simulink model "IEEE_39_bus_steady_state"  (R2021b)
settings: Solver=ode3  StartTime=0.0  StopTime=10  FixedStep=Ts  MaxStep=1/60  RelTol=1e-2  AbsTol=1e-1
PreLoadFcn:
  | Ts=50e-6; ssn_ieee39_params; dec=20;
InitFcn:
  | Ts=50e-6; ssn_ieee39_params; dec=20;
values from neighbouring files (symbols this model uses):
  f = 50    [ssn_ieee39_params_ctrl.m]
  fNom = f    (= 60)    [ssn_ieee39_params_ctrl.m]
  ILR = 5.02    [ssn_ieee39_params_ctrl.m]
  IQMIN = 0.1    [ssn_ieee39_params_ctrl.m]
  ISCLIM = 1    [ssn_ieee39_params_ctrl.m]
  ITFpu = 1.10    (= 1.1)    [ssn_ieee39_params_ctrl.m]
  K = 1    [ssn_ieee39_params_ctrl.m]
  K1 = 1    [ssn_ieee39_params_ctrl.m]
  K2 = 2    [ssn_ieee39_params_ctrl.m]
  KCL = 1.04    [ssn_ieee39_params_ctrl.m]
  KFB = 0    [ssn_ieee39_params_ctrl.m]
  KFF = 1    [ssn_ieee39_params_ctrl.m]
  KFIX = 1    [ssn_ieee39_params_ctrl.m]
  KG = 1    [ssn_ieee39_params_ctrl.m]
  KIA = 59.91    [ssn_ieee39_params_ctrl.m]
  KIOEX = 0.0303    [ssn_ieee39_params_ctrl.m]
  KIUEX = 0.0303    [ssn_ieee39_params_ctrl.m]
  KIUOEX = 1    [ssn_ieee39_params_ctrl.m]
  KIUUEX = 1    [ssn_ieee39_params_ctrl.m]
  KLR = 22.47    [ssn_ieee39_params_ctrl.m]
  KM = 1    [ssn_ieee39_params_ctrl.m]
  KOEL = 0.24    [ssn_ieee39_params_ctrl.m]
  Kp = 1    [ssn_ieee39_params_ctrl.m]
  KPA = 30    [ssn_ieee39_params_ctrl.m]
  KPOEL = 1    [ssn_ieee39_params_ctrl.m]
  KPOEX = 0    [ssn_ieee39_params_ctrl.m]
  KPUEX = 0    [ssn_ieee39_params_ctrl.m]
  KSCALE = 0.319    [ssn_ieee39_params_ctrl.m]
  KUF = 0    [ssn_ieee39_params_ctrl.m]
  KUI = 0.001    [ssn_ieee39_params_ctrl.m]
  KUL = 0.24    [ssn_ieee39_params_ctrl.m]
  s = 10    [ssn_ieee39_params_ctrl.m]
  TA = 0.01    [ssn_ieee39_params_ctrl.m]
  Tadj = 0    [ssn_ieee39_params_ctrl.m]
  taps = [1 1 1.07 1.07 1.009 1.025 1 1.025 1.025 1.025]*1    [ssn_ieee39_params_ctrl.m]
  TF = 0.02    [ssn_ieee39_params_ctrl.m]
  TG = 0.024    [ssn_ieee39_params_ctrl.m]
  TINV = 0    [ssn_ieee39_params_ctrl.m]
  TIT = 0.1    [ssn_ieee39_params_ctrl.m]
  TL_10_11_len = 14    [ssn_ieee39_params_ctrl.m]
  TL_10_13_len = 14    [ssn_ieee39_params_ctrl.m]
  TL_13_14_len = 32    [ssn_ieee39_params_ctrl.m]
  TL_14_15_len = 70    [ssn_ieee39_params_ctrl.m]
  TL_15_16_len = 31.5    [ssn_ieee39_params_ctrl.m]
  TL_16_17_len = 26    [ssn_ieee39_params_ctrl.m]
  TL_16_19_len = 61    [ssn_ieee39_params_ctrl.m]
  TL_16_21_len = 46    [ssn_ieee39_params_ctrl.m]
  TL_16_24_len = 15    [ssn_ieee39_params_ctrl.m]
  TL_17_18_len = 26    [ssn_ieee39_params_ctrl.m]
  TL_17_27_len = 59    [ssn_ieee39_params_ctrl.m]
  TL_1_2_len = 134    [ssn_ieee39_params_ctrl.m]
  TL_1_39_len = 105    [ssn_ieee39_params_ctrl.m]
  TL_21_22_len = 47    [ssn_ieee39_params_ctrl.m]
  TL_22_23_len = 33    [ssn_ieee39_params_ctrl.m]
  TL_24_23_len = 88    [ssn_ieee39_params_ctrl.m]
  TL_25_26_len = 101    [ssn_ieee39_params_ctrl.m]
  TL_26_27_len = 46.5    [ssn_ieee39_params_ctrl.m]
  TL_26_28_len = 151    [ssn_ieee39_params_ctrl.m]
  TL_26_29_len = 200    [ssn_ieee39_params_ctrl.m]
  TL_28_29_len = 48    [ssn_ieee39_params_ctrl.m]
  TL_2_25_len = 28    [ssn_ieee39_params_ctrl.m]
  TL_2_2_len = 49    [ssn_ieee39_params_ctrl.m]
  TL_3_18_len = 42    [ssn_ieee39_params_ctrl.m]
  TL_3_4_len = 53    [ssn_ieee39_params_ctrl.m]
  TL_4_14_len = 33    [ssn_ieee39_params_ctrl.m]
  TL_4_5_len = 32.5    [ssn_ieee39_params_ctrl.m]
  TL_5_6_len = 14    [ssn_ieee39_params_ctrl.m]
  TL_5_8_len = 32    [ssn_ieee39_params_ctrl.m]
  TL_6_11_len = 26.5    [ssn_ieee39_params_ctrl.m]
  TL_6_7_len = 25.5    [ssn_ieee39_params_ctrl.m]
  TL_7_8_len = 15    [ssn_ieee39_params_ctrl.m]
  TL_8_9_len = 93    [ssn_ieee39_params_ctrl.m]
  TL_9_39_len = 136    [ssn_ieee39_params_ctrl.m]
  TOEL = 5.00    (= 5)    [ssn_ieee39_params_ctrl.m]
  TQREF = 0    [ssn_ieee39_params_ctrl.m]
  TQSCL = 0.012    [ssn_ieee39_params_ctrl.m]
  Ts_PMU = 1/1000    (= 0.001)    [ssn_ieee39_params_ctrl.m]
  TU1 = 0    [ssn_ieee39_params_ctrl.m]
  TU2 = 0    [ssn_ieee39_params_ctrl.m]
  TU3 = 0    [ssn_ieee39_params_ctrl.m]
  TU4 = 0    [ssn_ieee39_params_ctrl.m]
  TUL = 0    [ssn_ieee39_params_ctrl.m]
  TUP = 0.050    (= 0.05)    [ssn_ieee39_params_ctrl.m]
  TUQ = .005    (= 0.005)    [ssn_ieee39_params_ctrl.m]
  TUV = 0.2    [ssn_ieee39_params_ctrl.m]
  VAAMAX = VAMAX    (= 7.05)    [ssn_ieee39_params_ctrl.m]
  VAMAX = 7.05    [ssn_ieee39_params_ctrl.m]
  VAMIN = -6.11    [ssn_ieee39_params_ctrl.m]
  VBMAX = 999    [ssn_ieee39_params_ctrl.m]
  VF = 0    [ssn_ieee39_params_ctrl.m]
  VFB = 0    [ssn_ieee39_params_ctrl.m]
  VMMAX = 7.05    [ssn_ieee39_params_ctrl.m]
  VMMIN = -6.11    [ssn_ieee39_params_ctrl.m]
  VOELmax1 = 0.2353    [ssn_ieee39_params_ctrl.m]
  VOELmax2 = 0.0    (= 0)    [ssn_ieee39_params_ctrl.m]
  VOELmin1 = -0.24    [ssn_ieee39_params_ctrl.m]
  VOELmin2 = -1.0    (= -1)    [ssn_ieee39_params_ctrl.m]
  VRMAX = 7.05    [ssn_ieee39_params_ctrl.m]
  VRMIN = -6.11    [ssn_ieee39_params_ctrl.m]
  VSCLmax = 0.20    (= 0.2)    [ssn_ieee39_params_ctrl.m]
  VSCLmin = -0.10    (= -0.1)    [ssn_ieee39_params_ctrl.m]
  VUELmax1 = 1    [ssn_ieee39_params_ctrl.m]
  VUELmax2 = 1    [ssn_ieee39_params_ctrl.m]
  VUELmin1 = -1    [ssn_ieee39_params_ctrl.m]
  VUELmin2 = -1    [ssn_ieee39_params_ctrl.m]
  VUImax = 1    [ssn_ieee39_params_ctrl.m]
  VUImin = -1    [ssn_ieee39_params_ctrl.m]
undefined symbols (not defined in the file or in its folder): D1, Delta, MOV_segment9, powergui
libraries: spsThreePhaseVIMeasurementLib x43, slpidlib x40, op_dpl_lib x32, powerlib_extras x30, simulink_extras x20, spsST2AModel x20, spsThreePhaseParallelRLCLoadLib x20, spsThreePhaseTransformerTwoWindingsLib x13, spsSynchronousMachinepuStandardLib x10, simulink x10, spsPower3phInstantaneousLib x10, spsThreePhasePISectionLineLib x4
(part 15 of 15)

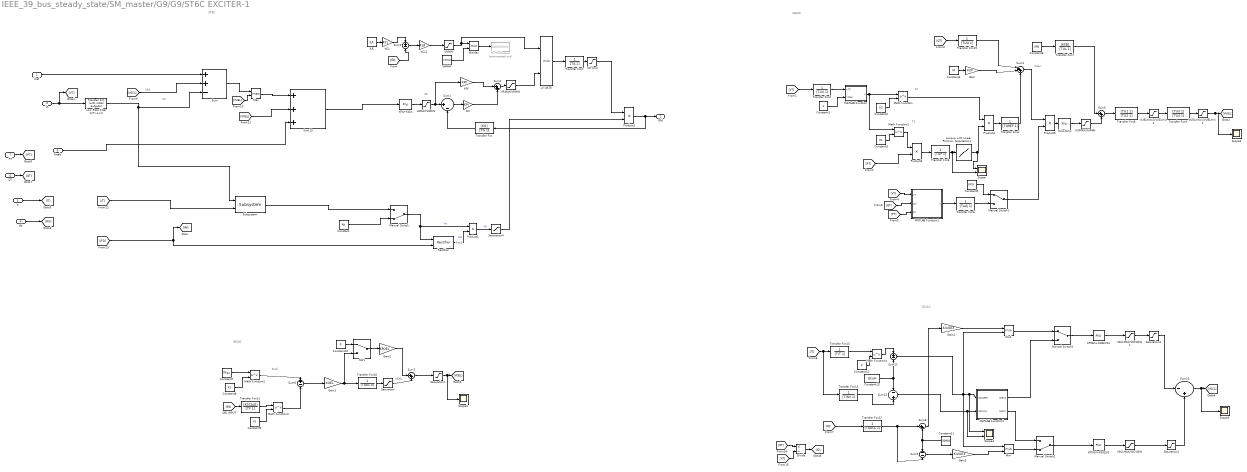
== system IEEE_39_bus_steady_state/SM_master/G9/G9/ST6C EXCITER-1 ==
  note: SCL1C
  note: OEL3C
  note: UEL2C
  note: VR0
  note: Fex0
  note: VA
  note: F2
  note: F1
  note: VUerr
  note: ST6C
  note: IFref
  note: VIOEL
  note: VC
  Vref : Inport
  Vt : Inport  Port=2
  It : Inport  Port=3
  Ifd : Inport  Port=4
  Vstab : Inport  Port=5
  QT : Inport  Port=6
  PT : Inport  Port=7
  Constant : Constant  Value=Kp
  Constant1 : Constant
  Constant10 : Constant  Value=0
  Constant11 : Constant  Value=IQMIN
  Constant12 : Constant  Value=K
  Constant13 : Constant  Value=ISCLIM
  Constant2 : Constant  Value=K2
  Constant3 : Constant  Value=K1
  Constant4 : Constant  Value=VF
  Constant5 : Constant  Value=KFIX
  Constant6 : Constant  Value=VFB
  Constant7 : Constant  Value=ITFpu
  Constant8 : Constant  Value=K1
  Constant9 : Constant  Value=K1
  Divide : Product  Inputs=*/
  Gain : Gain  Gain=KUF
  Gain1 : Gain  Gain=KOEL
  Gain2 : Gain  Gain=KPOEL
  Gain3 : Gain  Gain=KIUUEX
  Gain4 : Gain  Gain=KIUOEX
  ILR : Constant  Value=ILR
  KCL : Gain  Gain=KCL
  KCL1 : Gain  Gain=KLR
  KFF : Gain  Gain=KFF
  KM : Gain  Gain=KM
  KPA+KIA/s : slpidlib/PID Controller  Controller=PI  Form=Parallel  TimeDomain=Continuous-time  UseExternalTs=off  SampleTime=-1  IntegratorMethod=Forward Euler  FilterMethod=Forward Euler  ControllerParametersSource=internal  P=KPA  I=KIA  D=0  UseFilter=on  N=100  TunerSelectOption=Transfer Function Based (PID Tuner App)  InitialConditionSource=internal  InitialConditionForIntegrator=0  InitialConditionForFilter=0  DifferentiatorICPrevScaledInput=0  ExternalReset=none  TrackingMode=off  Kt=1  LimitOutput=off  SatLimitsSource=internal  UpperSaturationLimit=inf  LowerSaturationLimit=-inf  LinearizeAsGain=on  AntiWindupMode=none  Kb=1  POutMin=[]  POutMax=[]  IOutMin=[]  IOutMax=[]  DOutMin=[]  DOutMax=[]  NOutMin=[]  NOutMax=[]  SumOutMin=[]  SumOutMax=[]  SaturationOutMin=[]  SaturationOutMax=[]  PParamMin=[]  PParamMax=[]  IParamMin=[]  IParamMax=[]  DParamMin=[]  DParamMax=[]  NParamMin=[]  NParamMax=[]  KbParamMin=[]  KbParamMax=[]  KtParamMin=[]  KtParamMax=[]  KbOutMin=[]  KbOutMax=[]  KtOutMin=[]  KtOutMax=[]  IntegratorOutMin=[]  IntegratorOutMax=[]  FilterOutMin=[]  FilterOutMax=[]  SumI1OutMin=[]  SumI1OutMax=[]  SumI2OutMin=[]  SumI2OutMax=[]  SumI3OutMin=[]  SumI3OutMax=[]  SumI4OutMin=[]  SumI4OutMax=[]  SumDOutMin=[]  SumDOutMax=[]  DifferentiatorOutMin=[]  DifferentiatorOutMax=[]  FilterDiffOutCoefMin=[]  FilterDiffOutCoefMax=[]  ReciprocalOutMin=[]  ReciprocalOutMax=[]  SumDenOutMin=[]  SumDenOutMax=[]  SumNumOutMin=[]  SumNumOutMax=[]  DivideOutMin=[]  DivideOutMax=[]  UdiffTsProdOutMin=[]  UdiffTsProdOutMax=[]  NTsProdOutMin=[]  NTsProdOutMax=[]  UintegralTsProdOutMin=[]  UintegralTsProdOutMax=[]  UngainTsProdOutMin=[]  UngainTsProdOutMax=[]  FilterDenConstantOutDataTypeStr=Inherit: Inherit via back propagation  FilterDenConstantOutMin=[]  FilterDenConstantOutMax=[]  PCopyOutDataTypeStr=Inherit: Inherit via back propagation  PCopyOutMin=[]  PCopyOutMax=[]  NCopyOutDataTypeStr=Inherit: Inherit via back propagation  NCopyOutMin=[]  NCopyOutMax=[]  IntegratorContinuousStateAttributes=''  IntegratorStateMustResolveToSignalObject=off  IntegratorRTWStateStorageClass=Auto  FilterContinuousStateAttributes=''  FilterStateMustResolveToSignalObject=off  FilterRTWStateStorageClass=Auto  ParallelPVariant=InternalParameters  IdealPVariant=Disabled  IVariant=InternalParameters  DVariant=Disabled  IntegratorVariant=Continuous  SatVariant=Disabled  AWVariant=Passthrough  PCopyVariant=Disabled  TRVariant=Disabled  FdbkBlocksVariant=Forward  IdealPFdbkVariant=Disabled  SatFdbkVariant=Disabled  DerivativeFilterVariant=Disabled  NVariant=Disabled  NCopyVariant=Disabled_SignalSpec  FilterICVariant=Disabled  IntegratorICVariant=InternalICs  ExternalResetVariant=Disabled  TRSumVariant=Passthrough  SumFdbkVariant=Disabled  SumVariant=Sum_PI  TsampFilterVariant=InternalTs  TsampNgainVariant=Passthrough  TsampIntegralVariant=Passthrough  ExternalSaturationOutDataTypeStr=Inherit: Same as second input
  KPOEX+KIOEX/S1 : slpidlib/PID Controller  Controller=PI  Form=Parallel  TimeDomain=Continuous-time  UseExternalTs=off  SampleTime=-1  IntegratorMethod=Forward Euler  FilterMethod=Forward Euler  ControllerParametersSource=internal  P=KPOEX  I=KIOEX  D=0  UseFilter=on  N=100  TunerSelectOption=Transfer Function Based (PID Tuner App)  InitialConditionSource=internal  InitialConditionForIntegrator=0  InitialConditionForFilter=0  DifferentiatorICPrevScaledInput=0  ExternalReset=none  TrackingMode=off  Kt=1  LimitOutput=off  SatLimitsSource=internal  UpperSaturationLimit=inf  LowerSaturationLimit=-inf  LinearizeAsGain=on  AntiWindupMode=none  Kb=1  POutMin=[]  POutMax=[]  IOutMin=[]  IOutMax=[]  DOutMin=[]  DOutMax=[]  NOutMin=[]  NOutMax=[]  SumOutMin=[]  SumOutMax=[]  SaturationOutMin=[]  SaturationOutMax=[]  PParamMin=[]  PParamMax=[]  IParamMin=[]  IParamMax=[]  DParamMin=[]  DParamMax=[]  NParamMin=[]  NParamMax=[]  KbParamMin=[]  KbParamMax=[]  KtParamMin=[]  KtParamMax=[]  KbOutMin=[]  KbOutMax=[]  KtOutMin=[]  KtOutMax=[]  IntegratorOutMin=[]  IntegratorOutMax=[]  FilterOutMin=[]  FilterOutMax=[]  SumI1OutMin=[]  SumI1OutMax=[]  SumI2OutMin=[]  SumI2OutMax=[]  SumI3OutMin=[]  SumI3OutMax=[]  SumI4OutMin=[]  SumI4OutMax=[]  SumDOutMin=[]  SumDOutMax=[]  DifferentiatorOutMin=[]  DifferentiatorOutMax=[]  FilterDiffOutCoefMin=[]  FilterDiffOutCoefMax=[]  ReciprocalOutMin=[]  ReciprocalOutMax=[]  SumDenOutMin=[]  SumDenOutMax=[]  SumNumOutMin=[]  SumNumOutMax=[]  DivideOutMin=[]  DivideOutMax=[]  UdiffTsProdOutMin=[]  UdiffTsProdOutMax=[]  NTsProdOutMin=[]  NTsProdOutMax=[]  UintegralTsProdOutMin=[]  UintegralTsProdOutMax=[]  UngainTsProdOutMin=[]  UngainTsProdOutMax=[]  FilterDenConstantOutDataTypeStr=Inherit: Inherit via back propagation  FilterDenConstantOutMin=[]  FilterDenConstantOutMax=[]  PCopyOutDataTypeStr=Inherit: Inherit via back propagation  PCopyOutMin=[]  PCopyOutMax=[]  NCopyOutDataTypeStr=Inherit: Inherit via back propagation  NCopyOutMin=[]  NCopyOutMax=[]  IntegratorContinuousStateAttributes=''  IntegratorStateMustResolveToSignalObject=off  IntegratorRTWStateStorageClass=Auto  FilterContinuousStateAttributes=''  FilterStateMustResolveToSignalObject=off  FilterRTWStateStorageClass=Auto  ParallelPVariant=InternalParameters  IdealPVariant=Disabled  IVariant=InternalParameters  DVariant=Disabled  IntegratorVariant=Continuous  SatVariant=Disabled  AWVariant=Passthrough  PCopyVariant=Disabled  TRVariant=Disabled  FdbkBlocksVariant=Forward  IdealPFdbkVariant=Disabled  SatFdbkVariant=Disabled  DerivativeFilterVariant=Disabled  NVariant=Disabled  NCopyVariant=Disabled_SignalSpec  FilterICVariant=Disabled  IntegratorICVariant=InternalICs  ExternalResetVariant=Disabled  TRSumVariant=Passthrough  SumFdbkVariant=Disabled  SumVariant=Sum_PI  TsampFilterVariant=InternalTs  TsampNgainVariant=Passthrough  TsampIntegralVariant=Passthrough  ExternalSaturationOutDataTypeStr=Inherit: Same as second input
  KPUEX+KIUES/S : slpidlib/PID Controller  Controller=PI  Form=Parallel  TimeDomain=Continuous-time  UseExternalTs=off  SampleTime=-1  IntegratorMethod=Forward Euler  FilterMethod=Forward Euler  ControllerParametersSource=internal  P=KPUEX  I=KIUEX  D=0  UseFilter=on  N=100  TunerSelectOption=Transfer Function Based (PID Tuner App)  InitialConditionSource=internal  InitialConditionForIntegrator=0  InitialConditionForFilter=0  DifferentiatorICPrevScaledInput=0  ExternalReset=none  TrackingMode=off  Kt=1  LimitOutput=off  SatLimitsSource=internal  UpperSaturationLimit=inf  LowerSaturationLimit=-inf  LinearizeAsGain=on  AntiWindupMode=none  Kb=1  POutMin=[]  POutMax=[]  IOutMin=[]  IOutMax=[]  DOutMin=[]  DOutMax=[]  NOutMin=[]  NOutMax=[]  SumOutMin=[]  SumOutMax=[]  SaturationOutMin=[]  SaturationOutMax=[]  PParamMin=[]  PParamMax=[]  IParamMin=[]  IParamMax=[]  DParamMin=[]  DParamMax=[]  NParamMin=[]  NParamMax=[]  KbParamMin=[]  KbParamMax=[]  KtParamMin=[]  KtParamMax=[]  KbOutMin=[]  KbOutMax=[]  KtOutMin=[]  KtOutMax=[]  IntegratorOutMin=[]  IntegratorOutMax=[]  FilterOutMin=[]  FilterOutMax=[]  SumI1OutMin=[]  SumI1OutMax=[]  SumI2OutMin=[]  SumI2OutMax=[]  SumI3OutMin=[]  SumI3OutMax=[]  SumI4OutMin=[]  SumI4OutMax=[]  SumDOutMin=[]  SumDOutMax=[]  DifferentiatorOutMin=[]  DifferentiatorOutMax=[]  FilterDiffOutCoefMin=[]  FilterDiffOutCoefMax=[]  ReciprocalOutMin=[]  ReciprocalOutMax=[]  SumDenOutMin=[]  SumDenOutMax=[]  SumNumOutMin=[]  SumNumOutMax=[]  DivideOutMin=[]  DivideOutMax=[]  UdiffTsProdOutMin=[]  UdiffTsProdOutMax=[]  NTsProdOutMin=[]  NTsProdOutMax=[]  UintegralTsProdOutMin=[]  UintegralTsProdOutMax=[]  UngainTsProdOutMin=[]  UngainTsProdOutMax=[]  FilterDenConstantOutDataTypeStr=Inherit: Inherit via back propagation  FilterDenConstantOutMin=[]  FilterDenConstantOutMax=[]  PCopyOutDataTypeStr=Inherit: Inherit via back propagation  PCopyOutMin=[]  PCopyOutMax=[]  NCopyOutDataTypeStr=Inherit: Inherit via back propagation  NCopyOutMin=[]  NCopyOutMax=[]  IntegratorContinuousStateAttributes=''  IntegratorStateMustResolveToSignalObject=off  IntegratorRTWStateStorageClass=Auto  FilterContinuousStateAttributes=''  FilterStateMustResolveToSignalObject=off  FilterRTWStateStorageClass=Auto  ParallelPVariant=InternalParameters  IdealPVariant=Disabled  IVariant=InternalParameters  DVariant=Disabled  IntegratorVariant=Continuous  SatVariant=Disabled  AWVariant=Passthrough  PCopyVariant=Disabled  TRVariant=Disabled  FdbkBlocksVariant=Forward  IdealPFdbkVariant=Disabled  SatFdbkVariant=Disabled  DerivativeFilterVariant=Disabled  NVariant=Disabled  NCopyVariant=Disabled_SignalSpec  FilterICVariant=Disabled  IntegratorICVariant=InternalICs  ExternalResetVariant=Disabled  TRSumVariant=Passthrough  SumFdbkVariant=Disabled  SumVariant=Sum_PI  TsampFilterVariant=InternalTs  TsampNgainVariant=Passthrough  TsampIntegralVariant=Passthrough  ExternalSaturationOutDataTypeStr=Inherit: Same as second input
  KUI+KUI/s : slpidlib/PID Controller  Controller=PI  Form=Parallel  TimeDomain=Continuous-time  UseExternalTs=off  SampleTime=-1  IntegratorMethod=Forward Euler  FilterMethod=Forward Euler  ControllerParametersSource=internal  P=KUL  I=KUI  D=0  UseFilter=on  N=100  TunerSelectOption=Transfer Function Based (PID Tuner App)  InitialConditionSource=internal  InitialConditionForIntegrator=0  InitialConditionForFilter=0  DifferentiatorICPrevScaledInput=0  ExternalReset=none  TrackingMode=off  Kt=1  LimitOutput=off  SatLimitsSource=internal  UpperSaturationLimit=inf  LowerSaturationLimit=-inf  LinearizeAsGain=on  AntiWindupMode=none  Kb=1  POutMin=[]  POutMax=[]  IOutMin=[]  IOutMax=[]  DOutMin=[]  DOutMax=[]  NOutMin=[]  NOutMax=[]  SumOutMin=[]  SumOutMax=[]  SaturationOutMin=[]  SaturationOutMax=[]  PParamMin=[]  PParamMax=[]  IParamMin=[]  IParamMax=[]  DParamMin=[]  DParamMax=[]  NParamMin=[]  NParamMax=[]  KbParamMin=[]  KbParamMax=[]  KtParamMin=[]  KtParamMax=[]  KbOutMin=[]  KbOutMax=[]  KtOutMin=[]  KtOutMax=[]  IntegratorOutMin=[]  IntegratorOutMax=[]  FilterOutMin=[]  FilterOutMax=[]  SumI1OutMin=[]  SumI1OutMax=[]  SumI2OutMin=[]  SumI2OutMax=[]  SumI3OutMin=[]  SumI3OutMax=[]  SumI4OutMin=[]  SumI4OutMax=[]  SumDOutMin=[]  SumDOutMax=[]  DifferentiatorOutMin=[]  DifferentiatorOutMax=[]  FilterDiffOutCoefMin=[]  FilterDiffOutCoefMax=[]  ReciprocalOutMin=[]  ReciprocalOutMax=[]  SumDenOutMin=[]  SumDenOutMax=[]  SumNumOutMin=[]  SumNumOutMax=[]  DivideOutMin=[]  DivideOutMax=[]  UdiffTsProdOutMin=[]  UdiffTsProdOutMax=[]  NTsProdOutMin=[]  NTsProdOutMax=[]  UintegralTsProdOutMin=[]  UintegralTsProdOutMax=[]  UngainTsProdOutMin=[]  UngainTsProdOutMax=[]  FilterDenConstantOutDataTypeStr=Inherit: Inherit via back propagation  FilterDenConstantOutMin=[]  FilterDenConstantOutMax=[]  PCopyOutDataTypeStr=Inherit: Inherit via back propagation  PCopyOutMin=[]  PCopyOutMax=[]  NCopyOutDataTypeStr=Inherit: Inherit via back propagation  NCopyOutMin=[]  NCopyOutMax=[]  IntegratorContinuousStateAttributes=''  IntegratorStateMustResolveToSignalObject=off  IntegratorRTWStateStorageClass=Auto  FilterContinuousStateAttributes=''  FilterStateMustResolveToSignalObject=off  FilterRTWStateStorageClass=Auto  ParallelPVariant=InternalParameters  IdealPVariant=Disabled  IVariant=InternalParameters  DVariant=Disabled  IntegratorVariant=Continuous  SatVariant=Disabled  AWVariant=Passthrough  PCopyVariant=Disabled  TRVariant=Disabled  FdbkBlocksVariant=Forward  IdealPFdbkVariant=Disabled  SatFdbkVariant=Disabled  DerivativeFilterVariant=Disabled  NVariant=Disabled  NCopyVariant=Disabled_SignalSpec  FilterICVariant=Disabled  IntegratorICVariant=InternalICs  ExternalResetVariant=Disabled  TRSumVariant=Passthrough  SumFdbkVariant=Disabled  SumVariant=Sum_PI  TsampFilterVariant=InternalTs  TsampNgainVariant=Passthrough  TsampIntegralVariant=Passthrough  ExternalSaturationOutDataTypeStr=Inherit: Same as second input
  LV GATE : MinMax  Inputs=2
  Lookup with Linear Point-slope Interpolation1 : Lookup_n-D  NumberOfTableDimensions=1  BreakpointsForDimension1=[0 1]  BreakpointsForDimension2=[-0.29 0.58]  Table="[-0.29  0]"  InternalRulePriority=Speed  RndMeth=Simplest  InputSameDT=on
  Low Pass Filter 1/(Tr.s+1) : simulink_extras/Additional Linear/Transfer Fcn (with initial outputs)  N=1  D=[0.016 1]  Y0=Vt0  U0=Vt0
  MATLAB Function : MATLAB Function  TreatAsAtomicUnit=on
  MATLAB Function1 : MATLAB Function  TreatAsAtomicUnit=on
  MATLAB Function2 : MATLAB Function  TreatAsAtomicUnit=on
  Manual Switch : ManualSwitch  CurrentSetting=0
  Manual Switch1 : ManualSwitch
  Manual Switch2 : ManualSwitch  CurrentSetting=0
  Manual Switch3 : ManualSwitch
  Math Function{,1..4} (5 alike) : Math  Operator=pow  SignedPower=on  SaturateOnIntegerOverflow=on
  Max : MinMax  Function=max  Inputs=2
  Min : MinMax  Inputs=2
  Min1 : MinMax  Inputs=2
  MinMax : MinMax  Inputs=2
  Product{1..5} (5 alike) : Product  InputSameDT=on  RndMeth=Zero  SaturateOnIntegerOverflow=on  OutDataTypeStr=Inherit: Same as first input
  Rectifier : spsST2AModel/Continuous/Rectifier  Kc=Kc
      settings: SourceProductBaseCode=PS
  SW1 : ManualSwitch
  Saturation : Saturate  UpperLimit=VOELmax1  LowerLimit=VOELmin1
  Saturation1 : Saturate  UpperLimit=VOELmax2  LowerLimit=VOELmin2
  Saturation2 : Saturate  UpperLimit=inf  LowerLimit=0
  Saturation3 : Saturate  UpperLimit=inf  LowerLimit=0
  Saturation4 : Saturate  UpperLimit=VBMAX  LowerLimit=eps
  Scope : Scope  NumInputPorts=2
  Scope1 : Scope
  Scope2 : Scope
  Scope3 : Scope
  Scope4 : Scope  NumInputPorts=2
  Subsystem : spsST2AModel/Continuous/Subsystem  KI=KI  Kp=Kp
      settings: SourceProductBaseCode=PS
  Sum : Sum  Inputs=++-  InputSameDT=on  SaturateOnIntegerOverflow=on  OutDataTypeStr=Inherit: Same as first input
  Sum1 : Sum  Inputs=|+-
  Sum10 : Sum  Inputs=|-+
  Sum11 : Sum  Inputs=+-
  Sum12 : Sum  Inputs=-+
  Sum13 : Sum  Inputs=+++  InputSameDT=on  SaturateOnIntegerOverflow=on  OutDataTypeStr=Inherit: Same as first input
  Sum2 : Sum  Inputs=|++
  Sum3 : Sum  Inputs=+-
  Sum4 : Sum  Inputs=|--+
  Sum5 : Sum  Inputs=|++
  Sum6 : Sum  Inputs=+-
  Sum7 : Sum  Inputs=|++
  Sum8 : Sum  Inputs=|+-
  Sum9 : Sum  Inputs=--
  To Workspace : ToWorkspace  Commented=on  VariableName=VAAMAXSWa  SaveFormat=Timeseries  SampleTime=-1
  Transfer Fcn : TransferFcn  Numerator=[KG]  Denominator=[TG 1]
  Transfer Fcn1 : TransferFcn  Denominator=[TA 1]
  Transfer Fcn10 : TransferFcn  Denominator=[TOEL 0]
  Transfer Fcn11 : TransferFcn  Numerator=[KSCALE]  Denominator=[TF 1]
  Transfer Fcn12 : TransferFcn  Denominator=[TQSCL 1]
  Transfer Fcn13 : TransferFcn  Denominator=[TIT 1]
  Transfer Fcn14 : TransferFcn  Denominator=[TINV 1]
  Transfer Fcn15 : TransferFcn  Denominator=[TUQ 1]
  Transfer Fcn2 : TransferFcn  Denominator=[TUV 1]
  Transfer Fcn3 : TransferFcn  Denominator=[TUP 1]
  Transfer Fcn4 : TransferFcn  Denominator=[TQREF 1]
  Transfer Fcn6 : TransferFcn  Denominator=[Tadj 1]
  Transfer Fcn7 : TransferFcn  Numerator=[KFB]  Denominator=[TUL 1]
  Transfer Fcn8 : TransferFcn  Numerator=[TU1 1]  Denominator=[TU2 1]
  Transfer Fcn9 : TransferFcn  Numerator=[TU3 1]  Denominator=[TU4 1]
  "VAMAX " : Constant  Value=VAMAX
  VAMAX/VAMIN : Saturate  UpperLimit=VAAMAX  LowerLimit=VAMIN
  VM limit : Saturate  UpperLimit=VMMAX  LowerLimit=VMMIN
  VRMAX/VRMIN : Saturate  UpperLimit=VRMAX  LowerLimit=VRMIN
  VRMIN : Saturate  UpperLimit=inf  LowerLimit=VRMIN
  VSCLMAX/VSCLMIN : Saturate  UpperLimit=VSCLmax  LowerLimit=VSCLmin
  VSCLMAX/VSCLMIN1 : Saturate  UpperLimit=VSCLmax  LowerLimit=VSCLmin
  VUELmax1/VUELmin1 : Saturate  UpperLimit=VUELmax1  LowerLimit=VUELmin1
  "VUELmax2/VUELmin2 " : Saturate  UpperLimit=VUELmax2  LowerLimit=VUELmin2
  VUIMAX/VUIMIN : Saturate  UpperLimit=VUImax  LowerLimit=VUImin
  Efd : Outport  VectorParamsAs1DForOutWhenUnconnected=off
  wires:
  KCL1/1 -> VRMIN/1
  Saturation4/1 -> Product2/2
  PT/1 -> [PT]
  Divide/1 -> [IQ]
  [VT] -> Divide/2
  [QT] -> Divide/1
  QT/1 -> [QT]
  Ifd/1 -> [IFD]
  It/1 -> [IT]
  Sum13/1 -> KPA+KIA/s/1
  [VOEL] -> Sum13/2
  Max/1 -> Sum13/1
  [VUEL] -> Max/2
  Sum10/1 -> [VSCL], Scope3/1
  Sum12/1 -> MATLAB Function2/2(ISCLINV), Scope4/2
  Transfer Fcn14/1 -> Sum12/2
  Constant13/1 -> Sum11/2, Sum12/1
  Math Function4/1 -> Sum11/1
  Constant12/1 -> Math Function4/2
  Transfer Fcn13/1 -> Math Function4/1
  [IT] -> Transfer Fcn13/1, Transfer Fcn14/1
  Gain4/1 -> Min1/1
  Sum8/1 -> Gain4/1
  Sum11/1 -> MATLAB Function2/1(ISCLERR), Scope4/1, Min1/2, Min/1
  Min1/1 -> Manual Switch3/1
  MATLAB Function2/1(IOEX2) -> Manual Switch3/2
  Manual Switch3/1 -> KPOEX+KIOEX/S1/1
  VSCLMAX/VSCLMIN1/1 -> Saturation3/1
  KPOEX+KIOEX/S1/1 -> VSCLMAX/VSCLMIN1/1
  Saturation3/1 -> Sum10/1
  Saturation2/1 -> Sum10/2
  VSCLMAX/VSCLMIN/1 -> Saturation2/1
  KPUEX+KIUES/S/1 -> VSCLMAX/VSCLMIN/1
  Manual Switch2/1 -> KPUEX+KIUES/S/1
  MATLAB Function2/2(IUEX2) -> Manual Switch2/1
  Min/1 -> Manual Switch2/2
  Gain3/1 -> Min/2
  Sum9/1 -> Gain3/1
  Constant11/1 -> Sum9/1, Sum8/2
  Transfer Fcn12/1 -> Sum8/1, Sum9/2
  [IQ] -> Transfer Fcn12/1
  Saturation1/1 -> [VOEL], Scope1/1
  Sum7/1 -> Saturation1/1
  Constant10/1 -> SW1/1
  SW1/1 -> Gain2/1
  Gain2/1 -> Sum7/1
  Saturation/1 -> Sum7/2
  Transfer Fcn10/1 -> Saturation/1
  Transfer Fcn11/1 -> Math Function3/1
  Gain1/1 -> Transfer Fcn10/1, SW1/2
  Sum6/1 -> Gain1/1
  [Ifd] -> Transfer Fcn11/1
  Constant9/1 -> Math Function3/2
  Math Function3/1 -> Sum6/2
  Math Function2/1 -> Sum6/1
  Constant8/1 -> Math Function2/2
  Constant7/1 -> Math Function2/1
  VUELmax1/VUELmin1/1 -> [VUEL], Scope2/1
  Transfer Fcn9/1 -> VUELmax1/VUELmin1/1
  "VUELmax2/VUELmin2 "/1 -> Transfer Fcn9/1
  Transfer Fcn8/1 -> "VUELmax2/VUELmin2 "/1
  Sum5/1 -> Transfer Fcn8/1
  Constant6/1 -> Transfer Fcn7/1
  Transfer Fcn7/1 -> Sum5/1
  VUIMAX/VUIMIN/1 -> Sum5/2
  Manual Switch1/1 -> Product5/2
  Constant5/1 -> Manual Switch1/1
  Transfer Fcn6/1 -> Manual Switch1/2
  MATLAB Function1/1(u) -> Transfer Fcn6/1
  [QT] -> MATLAB Function1/2(QT)
  [PT] -> MATLAB Function1/3(PT)
  [VT] -> MATLAB Function1/1(VT)
  Product5/1 -> KUI+KUI/s/1
  Sum4/1 -> Product5/1
  Transfer Fcn15/1 -> Sum4/1
  [QT] -> Transfer Fcn15/1
  Gain/1 -> Sum4/2
  Constant4/1 -> Gain/1
  Transfer Fcn4/1 -> Sum4/3
  KUI+KUI/s/1 -> VUIMAX/VUIMIN/1
  Product4/1 -> Transfer Fcn4/1
  Lookup with Linear Point-slope Interpolation1/1 -> Product4/2, Scope/1
  Transfer Fcn3/1 -> Lookup with Linear Point-slope Interpolation1/1, Scope/2
  Product3/1 -> Transfer Fcn3/1
  [PT] -> Product3/2
  Math Function1/1 -> Product3/1
  Constant3/1 -> Math Function1/2
  Math Function/1 -> Product4/1
  Constant2/1 -> Math Function/2
  MATLAB Function/1(u) -> Math Function/1, Math Function1/1
  Constant1/1 -> MATLAB Function/2(Vbias)
  Transfer Fcn2/1 -> MATLAB Function/1(VTF)
  [VT] -> Transfer Fcn2/1
  LV GATE/1 -> Transfer Fcn1/1
  VAMAX/VAMIN/1 -> Sum1/1, KFF/1
  VRMIN/1 -> MinMax/1, LV GATE/1
  [Ifd] -> Sum3/2
  Sum3/1 -> KCL1/1
  ILR/1 -> KCL/1
  KM/1 -> Sum2/2
  KCL/1 -> Sum3/1
  KFF/1 -> Sum2/1
  Sum/1 -> Max/1
  VRMAX/VRMIN/1 -> LV GATE/2
  Product2/1 -> Transfer Fcn/1, Efd/1
  Low Pass Filter 1/(Tr.s+1)/1 -> Sum/3, Subsystem/1
  Sum1/1 -> KM/1
  Transfer Fcn/1 -> Sum1/2
  Constant/1 -> Manual Switch/2
  Vref/1 -> Sum/1
  [IT] -> Subsystem/2
  Vstab/1 -> Sum13/3
  Vt/1 -> Low Pass Filter 1/(Tr.s+1)/1, [VT]
  Sum2/1 -> VRMAX/VRMIN/1
  Rectifier/1 -> Product1/2  "Fex"
  [IFD] -> Rectifier/2, [Ifd]
  Product1/1 -> Saturation4/1  "VB"
  Manual Switch/1 -> Rectifier/1, Product1/1  "Ve"
  Subsystem/1 -> Manual Switch/1
  KPA+KIA/s/1 -> VAMAX/VAMIN/1
  [VSCL] -> Sum/2
  Transfer Fcn1/1 -> VM limit/1
  "VAMAX "/1 -> MinMax/2
  MinMax/1 -> To Workspace/1
  VM limit/1 -> Product2/1

== matlab function IEEE_39_bus_steady_state/SM_master/G10/G10/ST6C EXCITER-1/MATLAB Function ==
  data: VTF input; u output; Vbias input
function u = fcn(VTF,Vbias)
%#codegen
if VTF > 1
    u=VTF;
    
else if VTF > Vbias
        u=1;
    else
        u=VTF/Vbias
    end
end
u;

== matlab function IEEE_39_bus_steady_state/SM_master/G8/ G8/ST6C EXCITER-1/MATLAB Function1 ==
  data: VT input; u output; QT input; PT input
function u = fcn(VT,QT,PT)
Xq=0.474;
Kadj= (((VT*VT)/Xq)+QT)/(sqrt(((((VT*VT)/Xq)+QT)*(((VT*VT)/Xq)+QT))+(PT*PT)))
u= Kadj;

== matlab function IEEE_39_bus_steady_state/SM_master/G8/ G8/ST6C EXCITER-1/MATLAB Function2 ==
  data: ISCLERR input; IOEX2 output; ISCLINV input; IUEX2 output
function [IOEX2,IUEX2] = fcn(ISCLERR,ISCLINV)
%#codegen

IOEX2= 0;
IUEX2= 0;

== matlab function IEEE_39_bus_steady_state/SM_master/G2/G2/ST6C EXCITER-1/MATLAB Function1 ==
  data: VT input; u output; QT input; PT input
function u = fcn(VT,QT,PT)
Xq=0.474;
Kadj= (((VT*VT)/Xq)+QT)/(sqrt(((((VT*VT)/Xq)+QT)*(((VT*VT)/Xq)+QT))+(PT*PT)))
u= Kadj;

== matlab function IEEE_39_bus_steady_state/SM_master/G2/G2/ST6C EXCITER-1/MATLAB Function2 ==
  data: ISCLERR input; IOEX2 output; ISCLINV input; IUEX2 output
function [IOEX2,IUEX2] = fcn(ISCLERR,ISCLINV)
%#codegen

IOEX2= 0;
IUEX2= 0;

== matlab function IEEE_39_bus_steady_state/SM_master/G6/G6/ST6C EXCITER-1/MATLAB Function ==
  data: VTF input; u output; Vbias input
function u = fcn(VTF,Vbias)
%#codegen
if VTF > 1
    u=VTF;
    
else if VTF > Vbias
        u=1;
    else
        u=VTF/Vbias
    end
end
u;

== matlab function IEEE_39_bus_steady_state/SM_master/G6/G6/ST6C EXCITER-1/MATLAB Function1 ==
  data: VT input; u output; QT input; PT input
function u = fcn(VT,QT,PT)
Xq=0.474;
Kadj= (((VT*VT)/Xq)+QT)/(sqrt(((((VT*VT)/Xq)+QT)*(((VT*VT)/Xq)+QT))+(PT*PT)))
u= Kadj;

== matlab function IEEE_39_bus_steady_state/SM_master/G6/G6/ST6C EXCITER-1/MATLAB Function2 ==
  data: ISCLERR input; IOEX2 output; ISCLINV input; IUEX2 output
function [IOEX2,IUEX2] = fcn(ISCLERR,ISCLINV)
%#codegen

IOEX2= 0;
IUEX2= 0;

== matlab function IEEE_39_bus_steady_state/SM_master/G5/G5/ST6C EXCITER-1/MATLAB Function ==
  data: VTF input; u output; Vbias input
function u = fcn(VTF,Vbias)
%#codegen
if VTF > 1
    u=VTF;
    
else if VTF > Vbias
        u=1;
    else
        u=VTF/Vbias
    end
end
u;

== matlab function IEEE_39_bus_steady_state/SM_master/G5/G5/ST6C EXCITER-1/MATLAB Function1 ==
  data: VT input; u output; QT input; PT input
function u = fcn(VT,QT,PT)
Xq=0.474;
Kadj= (((VT*VT)/Xq)+QT)/(sqrt(((((VT*VT)/Xq)+QT)*(((VT*VT)/Xq)+QT))+(PT*PT)))
u= Kadj;

== matlab function IEEE_39_bus_steady_state/SM_master/G10/G10/ST6C EXCITER-1/MATLAB Function1 ==
  data: VT input; u output; QT input; PT input
function u = fcn(VT,QT,PT)
Xq=0.474;
Kadj= (((VT*VT)/Xq)+QT)/(sqrt(((((VT*VT)/Xq)+QT)*(((VT*VT)/Xq)+QT))+(PT*PT)))
u= Kadj;

== matlab function IEEE_39_bus_steady_state/SM_master/G5/G5/ST6C EXCITER-1/MATLAB Function2 ==
  data: ISCLERR input; IOEX2 output; ISCLINV input; IUEX2 output
function [IOEX2,IUEX2] = fcn(ISCLERR,ISCLINV)
%#codegen

IOEX2= 0;
IUEX2= 0;

== matlab function IEEE_39_bus_steady_state/SM_master/G4/G4/ST6C EXCITER-1/MATLAB Function ==
  data: VTF input; u output; Vbias input
function u = fcn(VTF,Vbias)
%#codegen
if VTF > 1
    u=VTF;
    
else if VTF > Vbias
        u=1;
    else
        u=VTF/Vbias
    end
end
u;

== matlab function IEEE_39_bus_steady_state/SM_master/G4/G4/ST6C EXCITER-1/MATLAB Function1 ==
  data: VT input; u output; QT input; PT input
function u = fcn(VT,QT,PT)
Xq=0.474;
Kadj= (((VT*VT)/Xq)+QT)/(sqrt(((((VT*VT)/Xq)+QT)*(((VT*VT)/Xq)+QT))+(PT*PT)))
u= Kadj;

== matlab function IEEE_39_bus_steady_state/SM_master/G4/G4/ST6C EXCITER-1/MATLAB Function2 ==
  data: ISCLERR input; IOEX2 output; ISCLINV input; IUEX2 output
function [IOEX2,IUEX2] = fcn(ISCLERR,ISCLINV)
%#codegen

IOEX2= 0;
IUEX2= 0;

== matlab function IEEE_39_bus_steady_state/SM_master/G7/G7/ST6C EXCITER-1/MATLAB Function ==
  data: VTF input; u output; Vbias input
function u = fcn(VTF,Vbias)
%#codegen
if VTF > 1
    u=VTF;
    
else if VTF > Vbias
        u=1;
    else
        u=VTF/Vbias
    end
end
u;

== matlab function IEEE_39_bus_steady_state/SM_master/G7/G7/ST6C EXCITER-1/MATLAB Function1 ==
  data: VT input; u output; QT input; PT input
function u = fcn(VT,QT,PT)
Xq=0.474;
Kadj= (((VT*VT)/Xq)+QT)/(sqrt(((((VT*VT)/Xq)+QT)*(((VT*VT)/Xq)+QT))+(PT*PT)))
u= Kadj;

== matlab function IEEE_39_bus_steady_state/SM_master/G7/G7/ST6C EXCITER-1/MATLAB Function2 ==
  data: ISCLERR input; IOEX2 output; ISCLINV input; IUEX2 output
function [IOEX2,IUEX2] = fcn(ISCLERR,ISCLINV)
%#codegen

IOEX2= 0;
IUEX2= 0;

== matlab function IEEE_39_bus_steady_state/SM_master/G3/G3/ST6C EXCITER-1/MATLAB Function ==
  data: VTF input; u output; Vbias input
function u = fcn(VTF,Vbias)
%#codegen
if VTF > 1
    u=VTF;
    
else if VTF > Vbias
        u=1;
    else
        u=VTF/Vbias
    end
end
u;

== matlab function IEEE_39_bus_steady_state/SM_master/G3/G3/ST6C EXCITER-1/MATLAB Function1 ==
  data: VT input; u output; QT input; PT input
function u = fcn(VT,QT,PT)
Xq=0.474;
Kadj= (((VT*VT)/Xq)+QT)/(sqrt(((((VT*VT)/Xq)+QT)*(((VT*VT)/Xq)+QT))+(PT*PT)))
u= Kadj;

== matlab function IEEE_39_bus_steady_state/SM_master/G3/G3/ST6C EXCITER-1/MATLAB Function2 ==
  data: ISCLERR input; IOEX2 output; ISCLINV input; IUEX2 output
function [IOEX2,IUEX2] = fcn(ISCLERR,ISCLINV)
%#codegen

IOEX2= 0;
IUEX2= 0;

== matlab function IEEE_39_bus_steady_state/SM_master/G10/G10/ST6C EXCITER-1/MATLAB Function2 ==
  data: ISCLERR input; IOEX2 output; ISCLINV input; IUEX2 output
function [IOEX2,IUEX2] = fcn(ISCLERR,ISCLINV)
%#codegen

IOEX2= 0;
IUEX2= 0;

== matlab function IEEE_39_bus_steady_state/SM_master/G9/G9/ST6C EXCITER-1/MATLAB Function ==
  data: VTF input; u output; Vbias input
function u = fcn(VTF,Vbias)
%#codegen
if VTF > 1
    u=VTF;
    
else if VTF > Vbias
        u=1;
    else
        u=VTF/Vbias
    end
end
u;

== matlab function IEEE_39_bus_steady_state/SM_master/G9/G9/ST6C EXCITER-1/MATLAB Function1 ==
  data: VT input; u output; QT input; PT input
function u = fcn(VT,QT,PT)
Xq=0.474;
Kadj= (((VT*VT)/Xq)+QT)/(sqrt(((((VT*VT)/Xq)+QT)*(((VT*VT)/Xq)+QT))+(PT*PT)))
u= Kadj;

== matlab function IEEE_39_bus_steady_state/SM_master/G9/G9/ST6C EXCITER-1/MATLAB Function2 ==
  data: ISCLERR input; IOEX2 output; ISCLINV input; IUEX2 output
function [IOEX2,IUEX2] = fcn(ISCLERR,ISCLINV)
%#codegen

IOEX2= 0;
IUEX2= 0;

== matlab function IEEE_39_bus_steady_state/SM_master/G1/G1/ST6C EXCITER-1/MATLAB Function ==
  data: VTF input; u output; Vbias input
function u = fcn(VTF,Vbias)
%#codegen
if VTF > 1
    u=VTF;
    
else if VTF > Vbias
        u=1;
    else
        u=VTF/Vbias
    end
end
u;

== matlab function IEEE_39_bus_steady_state/SM_master/G1/G1/ST6C EXCITER-1/MATLAB Function1 ==
  data: VT input; u output; QT input; PT input
function u = fcn(VT,QT,PT)
Xq=0.474;
Kadj= (((VT*VT)/Xq)+QT)/(sqrt(((((VT*VT)/Xq)+QT)*(((VT*VT)/Xq)+QT))+(PT*PT)))
u= Kadj;

== matlab function IEEE_39_bus_steady_state/SM_master/G1/G1/ST6C EXCITER-1/MATLAB Function2 ==
  data: ISCLERR input; IOEX2 output; ISCLINV input; IUEX2 output
function [IOEX2,IUEX2] = fcn(ISCLERR,ISCLINV)
%#codegen

IOEX2= 0;
IUEX2= 0;

== matlab function IEEE_39_bus_steady_state/SM_master/G2/G2/ST6C EXCITER-1/MATLAB Function ==
  data: VTF input; u output; Vbias input
function u = fcn(VTF,Vbias)
%#codegen
if VTF > 1
    u=VTF;
    
else if VTF > Vbias
        u=1;
    else
        u=VTF/Vbias
    end
end
u;

== matlab function IEEE_39_bus_steady_state/SM_master/G8/ G8/ST6C EXCITER-1/MATLAB Function ==
  data: VTF input; u output; Vbias input
function u = fcn(VTF,Vbias)
%#codegen
if VTF > 1
    u=VTF;
    
else if VTF > Vbias
        u=1;
    else
        u=VTF/Vbias
    end
end
u;
